simulink model "sym_assignment3"  (R2025b)
settings: Solver=FixedStepAuto  StartTime=0.0  StopTime=30  FixedStep=0.1  RelTol=1e-3
model workspace (MAT data in the model file):
  SL_ROS_VariableLengthArrays_MaxSizes.CommonInfo.ArrayTruncateAction = 'EmitWarning'
  SL_ROS_VariableLengthArrays_MaxSizes.MsgTypeMap = containers.Map
  SL_ROS_VariableLengthArrays_MaxSizes.MsgTypeMap.serialization.keys = {'sensor_msgs/Image', 'sensor_msgs/LaserScan'}
  SL_ROS_VariableLengthArrays_MaxSizes.MsgTypeMap.serialization.values{1}(1).PropertyName = 'data'
  SL_ROS_VariableLengthArrays_MaxSizes.MsgTypeMap.serialization.values{1}(1).DataType = 'uint8'
  SL_ROS_VariableLengthArrays_MaxSizes.MsgTypeMap.serialization.values{1}(1).MaxLength = 921600
  SL_ROS_VariableLengthArrays_MaxSizes.MsgTypeMap.serialization.values{1}(2).PropertyName = 'encoding'
  SL_ROS_VariableLengthArrays_MaxSizes.MsgTypeMap.serialization.values{1}(2).DataType = 'uint8'
  SL_ROS_VariableLengthArrays_MaxSizes.MsgTypeMap.serialization.values{1}(2).MaxLength = 128
  SL_ROS_VariableLengthArrays_MaxSizes.MsgTypeMap.serialization.values{2}(1).PropertyName = 'intensities'
  SL_ROS_VariableLengthArrays_MaxSizes.MsgTypeMap.serialization.values{2}(1).DataType = 'single'
  SL_ROS_VariableLengthArrays_MaxSizes.MsgTypeMap.serialization.values{2}(1).MaxLength = 360
  SL_ROS_VariableLengthArrays_MaxSizes.MsgTypeMap.serialization.values{2}(2).PropertyName = 'ranges'
  SL_ROS_VariableLengthArrays_MaxSizes.MsgTypeMap.serialization.values{2}(2).DataType = 'single'
  SL_ROS_VariableLengthArrays_MaxSizes.MsgTypeMap.serialization.values{2}(2).MaxLength = 360
  SL_ROS_VariableLengthArrays_MaxSizes.MsgTypeMap.serialization.uniformity = 0
  SL_ROS_VariableLengthArrays_MaxSizes.MsgTypeMap.serialization.keyType = 'char'
  SL_ROS_VariableLengthArrays_MaxSizes.MsgTypeMap.serialization.valueType = 'any'
values from neighbouring files (symbols this model uses):
  omega = 0.2    [ass_3.m]    (also in assignment_3.m)
undefined symbols (not defined in the file or in its folder): gray, Rec, SDTV, twist
libraries: ros2lib x7, simulink x2, visionstatistics x1, visionconversions x1, visiontextngfix x1
settings Model: Creator=flash  LastModifiedBy=matteocasazzaa

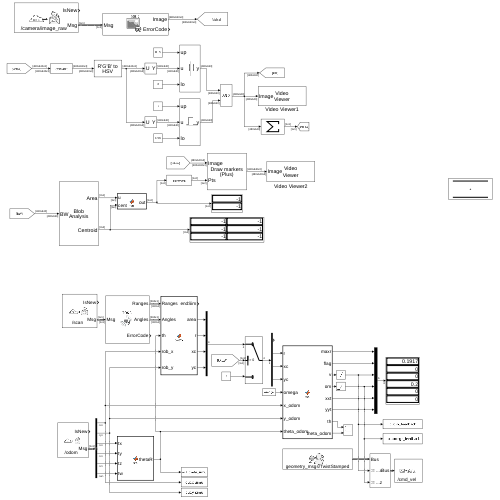
[thumbnail: Simulink's stored preview of the top-level diagram]
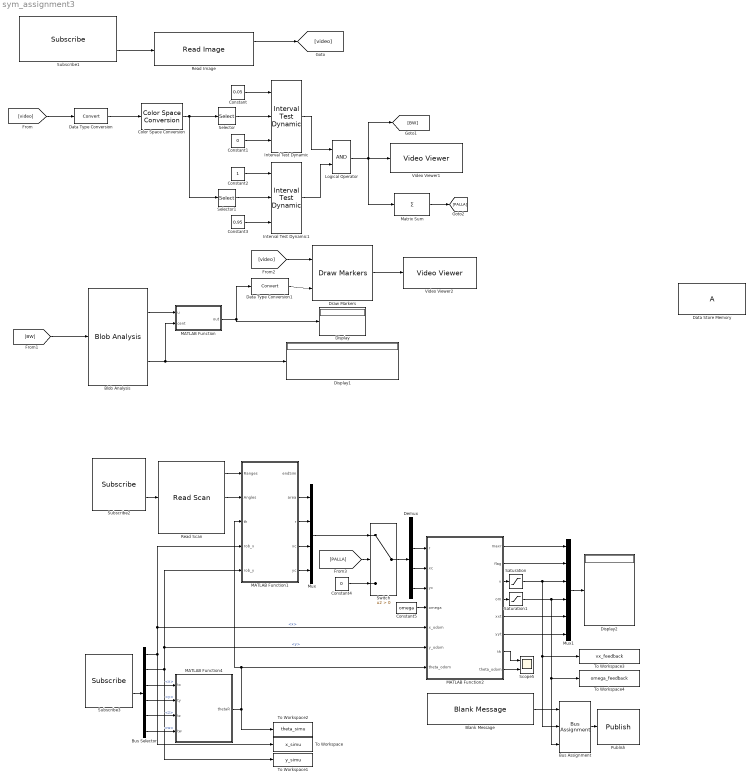
== system sym_assignment3 ==
  Blank Message : ros2lib/Blank Message  messageClass=Message  entityType=geometry_msgs/TwistStamped  messageType=geometry_msgs/TwistStamped  SampleTime=0.1
  Blob Analysis : visionstatistics/Blob Analysis  Tag=vipblks_row_conv  area=on  centroid=on  bBox=off  majorAxis=off  minorAxis=off  angle=off  eccentricity=off  equivDiameterSq=off  extent=off  perimeter=off  outDT=double  conn=8  isLabel=off  maxBlobs=3  warnIfNumBlobsExceeded=on  isCount=off  useMinArea=off  minArea=0  useMaxArea=off  maxArea=intmax('uint32')  excludeBorderBlob=off  isOutVarDim=off  isFill=on  fillValues=-1  roundingMode=Floor  overflowMode=off  prodOutputMode=Binary point scaling  prodOutputWordLength=32  prodOutputFracLength=16  accumMode=Binary point scaling  accumWordLength=32  accumFracLength=0  outputMode=Binary point scaling  outputWordLength=32  outputFracLength=16  firstCoeffMode=Binary point scaling  firstCoeffWordLength=16  firstCoeffFracLength=14  secondCoeffMode=Binary point scaling  secondCoeffWordLength=32  secondCoeffFracLength=16
  Bus Assignment : BusAssignment  AssignedSignals=twist.linear.x,twist.angular.z
  Bus Selector : BusSelector  OutputSignals=pose.pose.position.x,pose.pose.position.y,pose.pose.orientation.x,pose.pose.orientation.y,pose.pose.orientation.z,pose.pose.orientation.w
  Color Space Conversion : visionconversions/Color Space  Conversion  conversion=Obsolete  conversionActive=R'G'B' to HSV  wp_str=D65  rec=Rec. 601 (SDTV)  sys=1125/60/2:1  imagePorts=One multidimensional signal
  Constant : Constant  Value=0.05
  Constant1 : Constant  Value=0
  Constant2 : Constant
  Constant3 : Constant  Value=0.95
  Constant4 : Constant  Value=0
  Constant5 : Constant  Value=omega
  Data Store Memory : DataStoreMemory  WriteAfterWriteMsg=warning  ShowAdditionalParam=off
  Data Type Conversion : DataTypeConversion  SaturateOnIntegerOverflow=off  RndMeth=Floor
  Data Type Conversion1 : DataTypeConversion  SaturateOnIntegerOverflow=off  RndMeth=Floor
  Demux : Demux
  Display : Display
  Display1 : Display
  Display2 : Display
  Draw Markers : visiontextngfix/Draw Markers  shape=Plus  size=10  fill=off  fillClrSource=Specify via dialog  display=Black  intensity=200  color=[200 255 100]  opacity=0.6  viewport=Entire image  antialiasing=off  inType=Obsolete  imagePorts=One multidimensional signal  roundingMode=Floor  overflowMode=off  memoryMode=Specify word length  memoryWordLength=16  memoryFracLength=15  prodOutputMode=Binary point scaling  prodOutputWordLength=32  prodOutputFracLength=14
  Interval Test Dynamic : simulink/Logic and Bit Operations/Interval Test Dynamic  IntervalClosedRight=on  IntervalClosedLeft=on  OutDataTypeStr=boolean
  Interval Test Dynamic1 : simulink/Logic and Bit Operations/Interval Test Dynamic  IntervalClosedRight=on  IntervalClosedLeft=on  OutDataTypeStr=boolean
  Logical Operator : Logic  AllPortsSameDT=off  OutDataTypeStr=boolean
  MATLAB Function : MATLAB Function  TreatAsAtomicUnit=on
  MATLAB Function1 : MATLAB Function  TreatAsAtomicUnit=on
  MATLAB Function2 : MATLAB Function  TreatAsAtomicUnit=on
  MATLAB Function4 : MATLAB Function  TreatAsAtomicUnit=on
  Matrix Sum : Sum  Inputs=+
  Mux : Mux
  Mux1 : Mux  Inputs=6
  Publish : ros2lib/Publish  topicSource=Specify your own  topic=/cmd_vel  messageType=geometry_msgs/TwistStamped  QOSHistory=Keep last  QOSDepth=10  QOSReliability=Reliable  QOSDurability=Volatile  QOSDeadline=Inf  QOSLifespan=Inf  QOSLiveliness=Automatic  QOSLeaseDuration=Inf  QOSAvoidROSNamespaceConventions=off
  Read Image : ros2lib/Read Image  MaximumImageSize=[480, 640]  ImageEncoding=rgb8  ShowAlphaOutput=off  ShowErrorCodeOutput=on  VariableSizeOutputs=off
  Read Scan : ros2lib/Read Scan  MaximumArrayLength=360  ShowAnglesOutput=on  ShowIntensityOutput=off  ShowErrorCodeOutput=on  VariableSizeOutputs=on
  Saturation : Saturate  UpperLimit=0.4  LowerLimit=-0.4
  Saturation1 : Saturate  UpperLimit=0.2  LowerLimit=-0.2
  Scope5 : Scope  NumInputPorts=2
      settings: ActiveDisplayYMinimum=-0.7829413237520999  ActiveDisplayYMaximum=7.0464719137689009  DataLoggingVariableName=ScopeData5
  Selector : Selector  NumberOfDimensions=3  InputPortWidth=3  IndexOptions=Index vector (dialog),Index vector (dialog),Index vector (dialog)  Indices=[1:480],[1:640],1  OutputSizes=1,1,1
  Selector1 : Selector  NumberOfDimensions=3  InputPortWidth=3  IndexOptions=Index vector (dialog),Index vector (dialog),Index vector (dialog)  Indices=[1:480],[1:640],2  OutputSizes=1,1,1
  Subscribe1 : ros2lib/Subscribe  topicSource=Select from ROS network  topic=/camera/image_raw  messageType=sensor_msgs/Image  sampleTime=-1  QOSHistory=Keep last  QOSDepth=10  QOSReliability=Reliable  QOSDurability=Volatile  QOSDeadline=Inf  QOSLifespan=Inf  QOSLiveliness=Automatic  QOSLeaseDuration=Inf  QOSAvoidROSNamespaceConventions=off
  Subscribe2 : ros2lib/Subscribe  topicSource=Select from ROS network  topic=/scan  messageType=sensor_msgs/LaserScan  sampleTime=-1  QOSHistory=Keep last  QOSDepth=10  QOSReliability=Reliable  QOSDurability=Volatile  QOSDeadline=Inf  QOSLifespan=Inf  QOSLiveliness=Automatic  QOSLeaseDuration=Inf  QOSAvoidROSNamespaceConventions=off
  Subscribe3 : ros2lib/Subscribe  topicSource=Select from ROS network  topic=/odom  messageType=nav_msgs/Odometry  sampleTime=-1  QOSHistory=Keep last  QOSDepth=10  QOSReliability=Reliable  QOSDurability=Volatile  QOSDeadline=Inf  QOSLifespan=Inf  QOSLiveliness=Automatic  QOSLeaseDuration=Inf  QOSAvoidROSNamespaceConventions=off
  Switch : Switch  Criteria=u2 > Threshold  SaturateOnIntegerOverflow=off  InputSameDT=off
  To Workspace : ToWorkspace  VariableName=x_simu  SaveFormat=Timeseries  SampleTime=-1
  To Workspace1 : ToWorkspace  VariableName=y_simu  SaveFormat=Timeseries  SampleTime=-1
  To Workspace2 : ToWorkspace  VariableName=theta_simu  SaveFormat=Timeseries  SampleTime=-1
  To Workspace3 : ToWorkspace  VariableName=vx_feedback  SaveFormat=Timeseries  SampleTime=-1
  To Workspace4 : ToWorkspace  VariableName=omega_feedback  SaveFormat=Timeseries  SampleTime=-1
  Video Viewer1 : VideoViewer  FigPos=[67 1078 1854 935]
  Video Viewer2 : VideoViewer  colormapValue=gray(256)  FigPos=[67 1078 1854 935]
  wires:
  Read Scan/2 -> MATLAB Function1/2(Angles)
  Selector1/1 -> Interval Test Dynamic1/2
  Read Scan/1 -> MATLAB Function1/1(Ranges)
  Data Type Conversion/1 -> Color Space Conversion/1
  Interval Test Dynamic/1 -> Logical Operator/1
  Constant2/1 -> Interval Test Dynamic1/1
  Subscribe1/2 -> Read Image/1
  Blob Analysis/2 -> MATLAB Function/2(cent), Display1/1
  [BW] -> Blob Analysis/1
  Logical Operator/1 -> Video Viewer1/1, Matrix Sum/1, [BW]
  Color Space Conversion/1 -> Selector1/1, Selector/1
  Interval Test Dynamic1/1 -> Logical Operator/2
  Selector/1 -> Interval Test Dynamic/2
  Data Type Conversion1/1 -> Draw Markers/2
  Read Image/1 -> [video]
  MATLAB Function/1(out) -> Display/1, Data Type Conversion1/1
  Draw Markers/1 -> Video Viewer2/1
  Constant1/1 -> Interval Test Dynamic/3
  Subscribe2/2 -> Read Scan/1
  [video] -> Data Type Conversion/1
  Constant3/1 -> Interval Test Dynamic1/3
  [video] -> Draw Markers/1
  Blob Analysis/1 -> MATLAB Function/1(u)
  Constant/1 -> Interval Test Dynamic/1
  Matrix Sum/1 -> [PALLA]
  [PALLA] -> Switch/2
  Constant4/1 -> Switch/3
  MATLAB Function1/2(area) -> Mux/1
  MATLAB Function1/3(r) -> Mux/2
  MATLAB Function1/4(xc) -> Mux/3
  MATLAB Function1/5(yc) -> Mux/4
  Mux/1 -> Switch/1
  Switch/1 -> Demux/1
  Demux/2 -> MATLAB Function2/1(r)
  Mux1/1 -> Display2/1
  MATLAB Function2/1(maxr) -> Mux1/1
  Constant5/1 -> MATLAB Function2/4(omega)
  MATLAB Function2/2(flag) -> Mux1/2
  Bus Assignment/1 -> Publish/1
  Blank Message/1 -> Bus Assignment/1
  Demux/3 -> MATLAB Function2/2(xc)
  Demux/4 -> MATLAB Function2/3(yc)
  Subscribe3/2 -> Bus Selector/1
  Bus Selector/1 -> To Workspace/1, MATLAB Function2/5(x_odom), MATLAB Function1/4(rob_x)  "<x>"
  Bus Selector/2 -> To Workspace1/1, MATLAB Function1/5(rob_y), MATLAB Function2/6(y_odom)  "<y>"
  Bus Selector/3 -> MATLAB Function4/1(tx)  "<x>"
  Bus Selector/4 -> MATLAB Function4/2(ty)  "<y>"
  Bus Selector/5 -> MATLAB Function4/3(tz)  "<z>"
  Bus Selector/6 -> MATLAB Function4/4(tw)  "<w>"
  MATLAB Function2/3(v) -> Saturation/1
  MATLAB Function2/4(om) -> Saturation1/1
  Saturation/1 -> Mux1/3, To Workspace3/1, Bus Assignment/2
  Saturation1/1 -> Mux1/4, To Workspace4/1, Bus Assignment/3
  MATLAB Function2/5(xxt) -> Mux1/5
  MATLAB Function2/6(yyt) -> Mux1/6
  MATLAB Function4/1(thetaR) -> To Workspace2/1, MATLAB Function1/3(th), MATLAB Function2/7("theta_odom ")
  MATLAB Function2/8(theta_odom) -> Scope5/2
  MATLAB Function2/7(th) -> Scope5/1

== matlab function sym_assignment3/MATLAB Function1 ==
  data: Ranges input; endSim output; Angles input; area output; r output; xc output; yc output; th input; rob_x input; rob_y input
function [endSim,area,r,xc,yc] = plotXY(Ranges, Angles, th, rob_x, rob_y)

persistent hFig hScat        
persistent X_hist Y_hist ang_vect   

if isempty(hFig)
    hFig  = figure(1);       % crea la figura solo alla prima iterazione
    X_hist = [];
    Y_hist = [];
    ang_vect = [];
end


endSim = any(Ranges>0);

if endSim
    % x_lidar_global = rob_x + (l_x * cos(th) - l_y * sin(th));
    % y_lidar_global = rob_y + (l_x * sin(th) + l_y * cos(th));

    x = Ranges.*cos(Angles+th);
    y = Ranges.*sin(Angles+th);
    X = x(isfinite(x))+ rob_x;     %+ x_lidar_global;
    Y = y(isfinite(y))+ rob_y;     %+ y_lidar_global;

    % X = cos(th).*X + sin(th).*Y;
    % Y = sin(th).*X + cos(th).*Y;

    X_hist = [X_hist; X];
    Y_hist = [Y_hist; Y];

    % ang = atan(Y_hist./X_hist);
    ang=wrapTo2Pi(Angles+th);
    ang = ang(isfinite(x));
    ang_vect = [ang_vect; ang];
    ind = ang_vect>wrapTo2Pi(th) & ang_vect<wrapTo2Pi(th)+45/180*pi;
    X_if = X_hist(ind);
    Y_if = Y_hist(ind);

    A = [X_if Y_if ones(size(X_if))];
    B = X_if.^2 + Y_if.^2;

    C  = A\B;
    xc = C(1)/2;
    yc = C(2)/2;
    r  = sqrt(C(3) + xc^2 + yc^2);
    area = pi * r^2;

    %--- plotting incrementale ---
    figure(hFig);
    if isempty(hScat)
        hScat = plot(X_if, Y_if, '.', 'MarkerSize', 8); % primo plot
        hold('on');
        grid('on');
        axis('equal');
        ylim([-5 5]);
        xlim([-5 5]);
        xlabel('X'); ylabel('Y');
        title('Laser Scan cumulativo');
    else
        set(hScat, 'XData', X_hist, 'YData', Y_hist);        % aggiorna solo i dati
    end

    if length(X)>3
        plot(xc, yc, 'ro', 'MarkerSize', 8);
    end

else
    area = single(0.0);
    r    = single(0.0);
    xc   = single(0.0);
    yc   = single(0.0);
end

== matlab function sym_assignment3/MATLAB Function ==
  data: u input; out output; cent input
function out = fcn(u, cent)
[~,i] = max(u);

if ~isempty(i)
    out = cent(i,:);
else
    out = [0,0];
end

== matlab function sym_assignment3/MATLAB Function2 ==
  data: maxr output; flag output; r input; xc input; yc input; omega input; x_odom input; y_odom input; theta_odom input; v output; om output; xxt output; yyt output; th output; theta_odom output
function [maxr, flag, v, om, xxt, yyt, th, theta_odom] = fcn(r, xc, yc, omega, x_odom, y_odom, theta_odom)
v = 0;
om = omega;
flag = 0;

persistent max_r
persistent r_prev
persistent yy
persistent x_t y_t theta

if isempty(max_r) && isempty(r_prev) && isempty(yy)
    max_r = 0;
    r_prev = 0;
    yy = 0;
    x_t = 0;
    y_t = 0;
    theta = 0;
end

theta_odom = wrapTo2Pi(theta_odom);

alpha = 0.3;
rho = 0.5;
if yy == 1
    dy = y_odom - y_t;
    dx = x_odom - x_t;
    theta = pi + atan2(dy,dx);
    flag = 1;
    v = rho * sqrt(dy^2+dx^2);
    om = alpha*wrapToPi(theta - theta_odom);
end

theta_scan = atan((yc)/(xc));
% theta_abs = theta_scan + theta_odom;
dist = sqrt(xc^2 + yc^2);

if r_prev == 0 && r>0.75*max_r && r<1.25*max_r && flag==0
    x_t = -dist*cos(theta_scan) + x_odom;
    y_t = -dist*sin(theta_scan) + y_odom;
    dy = y_odom - y_t;
    dx = x_odom - x_t;
    theta = pi + atan(dy/ dx);
    flag = 1;
    v = rho * sqrt(dy^2+dx^2);
    om = alpha*wrapToPi(theta - theta_odom);
end

if r<0.5
    if r>max_r
        max_r = r;
    end
else
    r = 0;
end

maxr = max_r;
r_prev = r;
yy = flag;
xxt = x_t;
yyt = y_t;
th = theta;

== matlab function sym_assignment3/MATLAB Function4 ==
  data: tx input; thetaR output; ty input; tz input; tw input
function thetaR = fcn(tx, ty, tz, tw)
q = [tw, tx, ty, tz];
eul = quat2eul(q, 'ZYX');
thetaR = eul(1);
end
